simulink model "Laborversuch_2_Aufgabe_1"  (R2023b)
settings: Solver=VariableStepAuto  StartTime=0.0  StopTime=70  RelTol=1e-3
values from neighbouring files (symbols this model uses):
  AB = 0.0226    [Versuch_1_parameter.m]
  KR = 0.002    [Versuch_1_parameter.m]
settings Model: Creator=danie  LastModifiedBy=danie

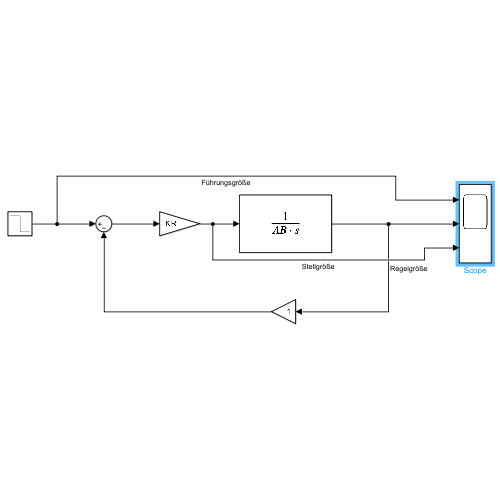
[thumbnail: Simulink's stored preview of the top-level diagram]
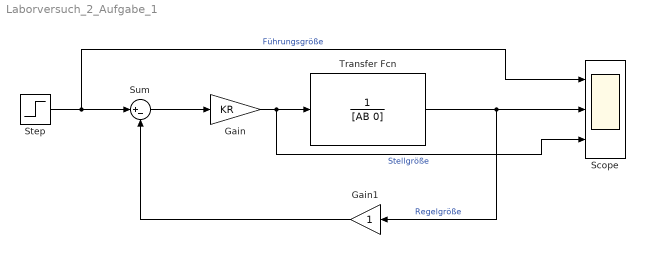
== system Laborversuch_2_Aufgabe_1 ==
  Gain : Gain  Gain=KR
  Gain1 : Gain
  Scope : Scope  NumInputPorts=3
  Step : Step  Time=70  Before=0.1  After=0  SampleTime=0
  Sum : Sum  Inputs=|+-
  Transfer Fcn : TransferFcn  Denominator=[AB 0]
  wires:
  Sum/1 -> Gain/1
  Gain/1 -> Scope/3, Transfer Fcn/1  "Stellgröße"
  Gain1/1 -> Sum/2
  Transfer Fcn/1 -> Gain1/1, Scope/2  "Regelgröße"
  Step/1 -> Scope/1, Sum/1  "Führungsgröße"
